simulink model "decode"  (R2021a)
settings: Solver=VariableStepAuto  StartTime=0.0  StopTime=36e-5  RelTol=1e-3
settings Model: Creator=sbetu  LastModifiedBy=sbetu

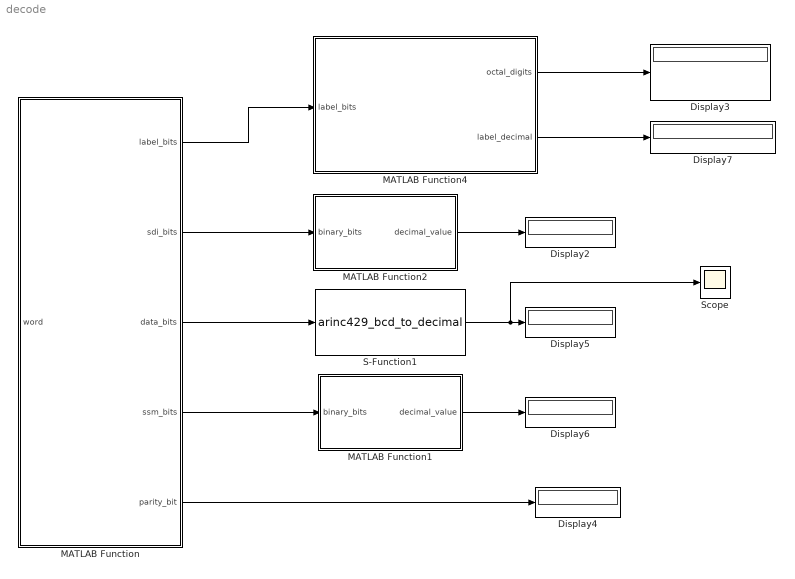
== system decode ==
  Display{2..7} (6 alike) : Display
  MATLAB Function : MATLAB Function  TreatAsAtomicUnit=on
  MATLAB Function1 : MATLAB Function  TreatAsAtomicUnit=on
  MATLAB Function2 : MATLAB Function  TreatAsAtomicUnit=on
  MATLAB Function4 : MATLAB Function  TreatAsAtomicUnit=on
  S-Function1 : S-Function  FunctionName=arinc429_bcd_to_decimal  SFunctionDeploymentMode=off  EnableBusSupport=off
  Scope : Scope
  wires:
  MATLAB Function/3(data_bits) -> S-Function1/1
  MATLAB Function4/2(label_decimal) -> Display7/1
  MATLAB Function1/1(decimal_value) -> Display6/1
  MATLAB Function/5(parity_bit) -> Display4/1
  MATLAB Function4/1(octal_digits) -> Display3/1
  MATLAB Function/2(sdi_bits) -> MATLAB Function2/1(binary_bits)
  MATLAB Function/4(ssm_bits) -> MATLAB Function1/1(binary_bits)
  S-Function1/1 -> Scope/1, Display5/1
  MATLAB Function/1(label_bits) -> MATLAB Function4/1(label_bits)
  MATLAB Function2/1(decimal_value) -> Display2/1
  ? -> MATLAB Function/1(word)

== matlab function decode/MATLAB Function ==
  data: word input; label_bits output; sdi_bits output; data_bits output; ssm_bits output; parity_bit output
function [label_bits, sdi_bits, data_bits, ssm_bits, parity_bit] = arinc_bit_extractor(word)
% ARINC 429 Raw Bit Extractor for Simulink MATLAB Function Block
% Sadece bitleri çıkarır, hiçbir işlem yapmaz
% Input:  word - uint32 ARINC 429 word
% Outputs: label_bits  - [8x1] uint8 Label bits (MSB'den LSB'ye)
%          sdi_bits    - [2x1] uint8 SDI bits
%          data_bits   - [19x1] uint8 Data bits  
%          ssm_bits    - [2x1] uint8 SSM bits
%          parity_bit  - uint8 Parity bit

    % Initialize outputs
    label_bits = zeros(8, 1, 'uint8');
    sdi_bits = zeros(2, 1, 'uint8');
    data_bits = zeros(19, 1, 'uint8');
    ssm_bits = zeros(2, 1, 'uint8');
    parity_bit = uint8(0);
    
    % Extract all 32 bits from word (LSB first)
    bits = zeros(32, 1, 'uint8');
    for k = 1:32
        bits(k) = uint8(bitget(word, k));
    end
    
    % Extract components (flip to match your original format)
    % ARINC 429 Format: [Label(8)] [SDI(2)] [Data(19)] [SSM(2)] [Parity(1)]
    
    % Label (bits 1-8, flip to MSB first)
    label_bits = flipud(bits(1:8));
    
    % SDI (bits 9-10, flip to MSB first)  
    sdi_bits = flipud(bits(9:10));
    
    % Data (bits 11-29, flip to MSB first)
    data_bits = flipud(bits(11:29));
    
    % SSM (bits 30-31, flip to MSB first)
    ssm_bits = flipud(bits(30:31));
    
    % Parity (bit 32)
    parity_bit = bits(32);
end

% Alternatif: Tek bir bileşen çıkaran fonksiyon
function bits_out = extract_single_component(word, component_type)
% Tek bir bileşenin bitlerini çıkarır
% Input:  word - uint32 ARINC 429 word
%         component_type - uint8 (1=Label, 2=SDI, 3=Data, 4=SSM, 5=Parity)
% Output: bits_out - uint8 array (boyut component'e göre değişir)

    % Extract all 32 bits
    bits = zeros(32, 1, 'uint8');
    for k = 1:32
        bits(k) = uint8(bitget(word, k));
    end
    
    if component_type == 1 % Label
        bits_out = flipud(bits(1:8));
    elseif component_type == 2 % SDI
        bits_out = flipud(bits(9:10));
    elseif component_type == 3 % Data
        bits_out = flipud(bits(11:29));
    elseif component_type == 4 % SSM
        bits_out = flipud(bits(30:31));
    elseif component_type == 5 % Parity
        bits_out = bits(32);
    else
        bits_out = uint8(0);
    end
end

== matlab function decode/MATLAB Function1 ==
  data: binary_bits input; decimal_value output

function decimal_value = binary_to_decimal(binary_bits)
% Binary to Decimal Converter for Simulink MATLAB Function Block
% Input:  binary_bits - [Nx1] uint8 binary array (MSB first)
% Output: decimal_value - double decimal value

    decimal_value = double(0);
    n = length(binary_bits);
    
    % Convert binary array to decimal
    % MSB first format: binary_bits(1) is most significant bit
    for i = 1:n
        if binary_bits(i) == 1
            decimal_value = decimal_value + 2^(n-i);
        end
    end
end

== matlab function decode/MATLAB Function2 ==
  data: binary_bits input; decimal_value output

function decimal_value = binary_to_decimal(binary_bits)
% Binary to Decimal Converter for Simulink MATLAB Function Block
% Input:  binary_bits - [Nx1] uint8 binary array (MSB first)
% Output: decimal_value - double decimal value

    decimal_value = double(0);
    n = length(binary_bits);
    
    % Convert binary array to decimal
    % MSB first format: binary_bits(1) is most significant bit
    for i = 1:n
        if binary_bits(i) == 1
            decimal_value = decimal_value + 2^(n-i);
        end
    end
end

== matlab function decode/MATLAB Function4 ==
  data: label_bits input; octal_digits output; label_decimal output
function [octal_digits, label_decimal] = arinc_label_bits_to_octal_decimal(label_bits)
% ARINC 429 Label: 8 bitlik giriş (MSB başta, LSB sonda)
% Çıkış: octal_digits = [3x1], label_decimal = decimal (0-255)

    % Bitleri tersle: LSB başa gelecek şekilde (ARINC 429'daki fiziksel yerleşime göre)
    bits = flip(label_bits(:)); % [8x1], bits(1) = LSB

    % 2+3+3 gruplara ayır
    group1 = bits(1:2);      % En anlamlı (2 bit)
    group2 = bits(3:5);      % Orta (3 bit)
    group3 = bits(6:8);      % En az anlamlı (3 bit)

    % Octal basamaklarını bul
    d1 = group1(1)*2 + group1(2)*1;                             % 2 bit
    d2 = group2(1)*4 + group2(2)*2 + group2(3)*1;               % 3 bit
    d3 = group3(1)*4 + group3(2)*2 + group3(3)*1;               % 3 bit

    octal_digits = [d1; d2; d3];

    % Decimal değeri hesapla (basamakları birleştirerek)
    label_decimal = d1*64 + d2*8 + d3;

    % Alternatif olarak: Doğrudan binary->decimal
    % label_decimal = sum(bits' .* 2.^(7:-1:0));
end
